simulink model "zftz"  (Simulink 5.0)
settings: Solver=ode5  StartTime=0.0  StopTime=0.5  FixedStep=0.00001  RelTol=1e-3
settings Model: LastModifiedBy=Administrator

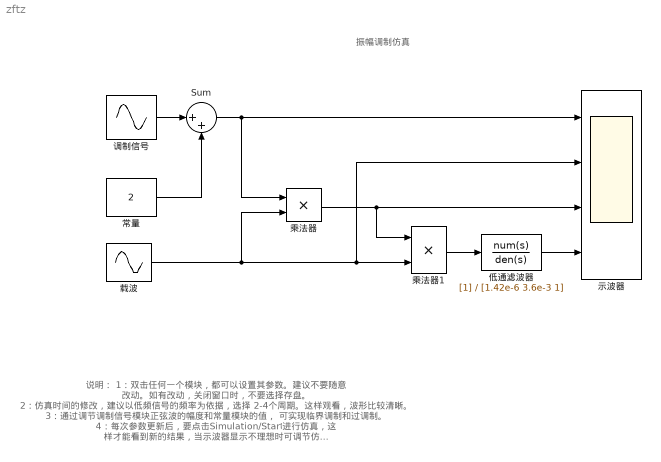
== system zftz ==
  note: 说明：
      | 1：双击任何一个模块，都可以设置其参数。建议不要随意
      |       改动。如有改动，关闭窗口时，不要选择存盘。
      | 2：仿真时间的修改，建议以低频信号的频率为依据，选择
      |       2-4个周期。这样观看，波形比较清晰。
      | 3：通过调节调制信号模块正弦波的幅度和常量模块的值，
      |       可实现临界调制和过调制。
      | 4：每次参数更新后，要点击Simulation/Start进行仿真，这
      |       样才能看到新的结果，当示波器显示不理想时可调节仿
      |       真时间，载波频率。当示波器Autoscale处于可用状态，
      |       可点击之。
  note: 振幅调制仿真
  Sum : Sum  Inputs=|++  SaturateOnIntegerOverflow=on
  常量 : Constant  Value=2
  乘法器 : Product  SaturateOnIntegerOverflow=on
  乘法器1 : Product  SaturateOnIntegerOverflow=on
  低通滤波器 : TransferFcn  Denominator=[1.42e-6 3.6e-3 1]
  调制信号 : Sin  Frequency=200  SampleTime=0
  示波器 : Scope  NumInputPorts=4
      settings: YMin=-5~-5~-5~-5  YMax=5~5~5~5
  载波 : Sin  Amplitude=2  Frequency=10000  Phase=90  SampleTime=0
  wires:
  载波/1 -> 乘法器/2, 示波器/2, 乘法器1/2
  乘法器/1 -> 示波器/3, 乘法器1/1
  调制信号/1 -> Sum/1
  常量/1 -> Sum/2
  Sum/1 -> 乘法器/1, 示波器/1
  乘法器1/1 -> 低通滤波器/1
  低通滤波器/1 -> 示波器/4
